simulink model "pressure"  (R2023b)
settings: Solver=FixedStepAuto  StartTime=0.0  StopTime=inf  RelTol=1e-3  EnableMultiTasking=on
PreLoadFcn:
  | a = 1;
InitFcn:
  | a = 1;
libraries: dspsigops x4, dspstat3 x3, simulink x2, bbblueSensorLib x1, dspfdesign x1
settings Model: SimulationMode=external  ExtModeTrigDuration=100  Creator=felih  LastModifiedBy=felih
settings SolverCC: PositivePriorityOrder=on
settings OptimizationCC: EnhancedBackFolding=on  PassReuseOutputArgsAs=Individual arguments  ZeroExternalMemoryAtStartup=off  ZeroInternalMemoryAtStartup=off  MaxStackSize=64  OptimizeBlockOrder=speed  DifferentSizesBufferReuse=on  OptimizationCustomize=off  EfficientTunableParamExpr=on
settings DebuggingCC: ParameterTunabilityLossMsg=error
settings HardwareCC: ProdBitPerPointer=32  ProdBitPerSizeT=32  ProdBitPerPtrDiffT=32  ProdLargestAtomicInteger=Long  ProdLargestAtomicFloat=Double  ProdWordSize=32  ProdHWDeviceType=ARM Compatible->ARM Cortex
settings SFSimCC: MATLABDynamicMemAlloc=off
settings RTWCC: Description=Embedded Coder  SystemTargetFile=ert.tlc  HardwareBoard=BeagleBone Blue  TLCOptions="-aInlineSetEventsForThisBaseRateFcn=TLC_FALSE -aSuppressMultiTaskScheduler=TLC_FALSE  -aRateBasedStepFcn=0"  TemplateMakefile=ert_default_tmf  Toolchain=GNU GCC BeagleBone Blue
settings CodeAppCC: ForceParamTrailComments=on  IgnoreCustomStorageClasses=off  OperatorAnnotations=on  SimulinkDataObjDesc=on  SFDataObjDesc=on  InsertBlockDesc=on
settings ERTTargetCC: SupportContinuousTime=on  SupportVariableSizeSignals=on  ExtMode=on  ExtModeMexArgs='192.168.7.2' 0 17725

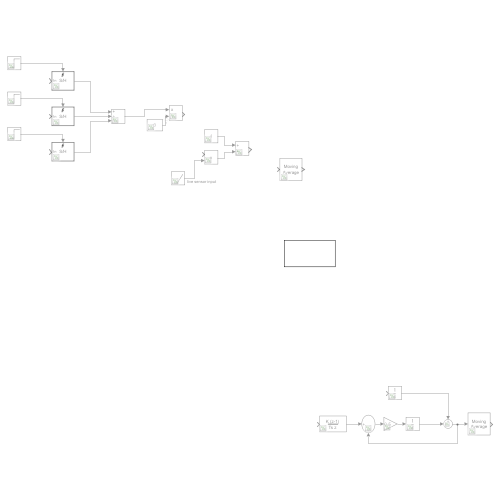
[thumbnail: Simulink's stored preview of the top-level diagram]
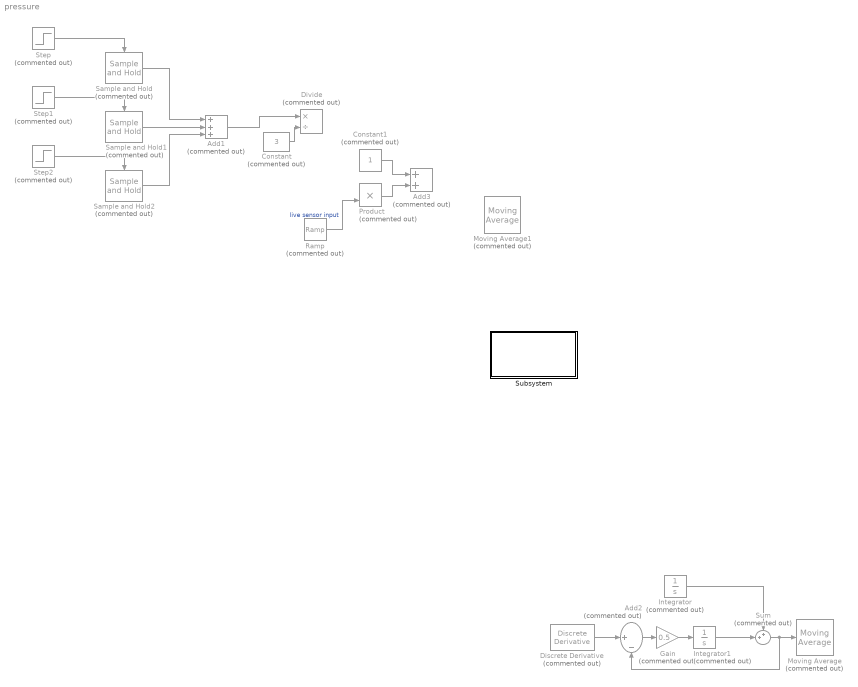
== system pressure ==
  Add1 : Sum  Commented=on  Inputs=+++
  Add2 : Sum  Commented=on  Inputs=|+-
  Add3 : Sum  Commented=on
  Constant : Constant  Commented=on  Value=3
  Constant1 : Constant  Commented=on
  Discrete Derivative : simulink/Discrete/Discrete Derivative  Commented=on  gainval=2  ICPrevScaledInput=0.0  OutMin=[]  OutMax=[]  OutDataType=fixdt(1, 16)  OutScaling=2^-10  DoSatur=off
  Divide : Product  Commented=on  Inputs=*/  RndMeth=Zero  SaturateOnIntegerOverflow=on
  Gain : Gain  Commented=on  Gain=0.5
  Integrator : Integrator  Commented=on
  Integrator1 : Integrator  Commented=on
  Moving Average : dspstat3/Moving Average  Commented=on  Method=Exponential weighting  ForgettingFactorPort=off  SpecifyWindowLength=on  WindowLength=10  OverlapLength=5  AllowArbitraryInputLength=off  ForgettingFactor=0.5  SimulateUsing=Code generation
  Moving Average1 : dspstat3/Moving Average  Commented=on  Method=Exponential weighting  ForgettingFactorPort=off  SpecifyWindowLength=on  WindowLength=10  OverlapLength=5  AllowArbitraryInputLength=on  ForgettingFactor=0.9  SimulateUsing=Code generation
  Product : Product  Commented=on
  Ramp : simulink/Sources/Ramp  Commented=on  slope=1  start=0  InitialOutput=0
  Sample and Hold : dspsigops/Sample and Hold  Commented=on  trig=Rising edge  initCond=0  latchinput=off
  Sample and Hold1 : dspsigops/Sample and Hold  Commented=on  trig=Rising edge  initCond=0  latchinput=off
  Sample and Hold2 : dspsigops/Sample and Hold  Commented=on  trig=Rising edge  initCond=0  latchinput=off
  Step : Step  Commented=on  SampleTime=0
  Step1 : Step  Commented=on  Time=1.1  SampleTime=0
  Step2 : Step  Commented=on  Time=0.9  SampleTime=0
  Subsystem : Subsystem
  Sum : Sum  Commented=on  Inputs=++|
  wires:
  Sample and Hold/1 -> Add1/1
  Sample and Hold1/1 -> Add1/2
  Step/1 -> Sample and Hold/Trigger
  Sample and Hold2/1 -> Add1/3
  Step1/1 -> Sample and Hold1/Trigger
  Step2/1 -> Sample and Hold2/Trigger
  Constant/1 -> Divide/2
  Add1/1 -> Divide/1
  Discrete Derivative/1 -> Add2/1
  Integrator1/1 -> Sum/2
  Integrator/1 -> Sum/1
  Add2/1 -> Gain/1
  Sum/1 -> Moving Average/1, Add2/2
  Gain/1 -> Integrator1/1
  Product/1 -> Add3/2
  Ramp/1 -> Product/2  "live sensor input"
  Constant1/1 -> Add3/1

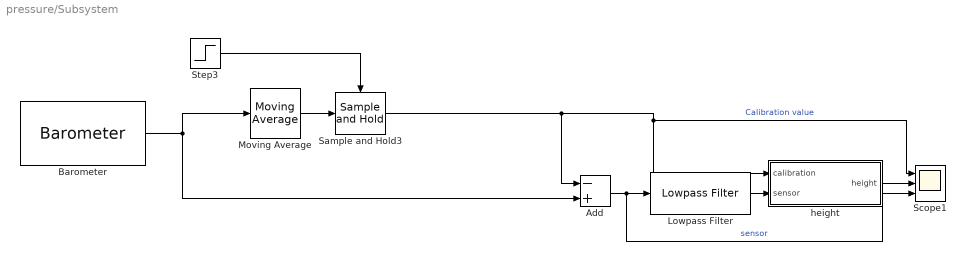
== system pressure/Subsystem ==
  Add : Sum  Inputs=-+
  Barometer : bbblueSensorLib/Barometer  OSRSelection=16  IIRFilterCoeff=2  SampleTime=0.01
  Lowpass Filter : dspfdesign/Lowpass Filter  FilterType=FIR  DesignForMinimumOrder=on  FilterOrder=50  PassbandFrequency=500  StopbandFrequency=800  PassbandRipple=0.1  StopbandAttenuation=80  SampleRateMode=Specify on dialog  SampleRate=44100  SimulateUsing=Interpreted execution  roundingMode=Floor  coeffsDataTypeStr=fixdt(1,16)
  Moving Average : dspstat3/Moving Average  Method=Exponential weighting  ForgettingFactorPort=off  SpecifyWindowLength=on  WindowLength=4  OverlapLength=3  AllowArbitraryInputLength=off  ForgettingFactor=1.0  SimulateUsing=Code generation
  Sample and Hold3 : dspsigops/Sample and Hold  trig=Rising edge  initCond=0  latchinput=off
  Scope1 : Scope  NumInputPorts=3
  Step3 : Step  Time=2  SampleTime=0
  height : MATLAB Function  TreatAsAtomicUnit=on
  wires:
  Add/1 -> Lowpass Filter/1, Scope1/3  "sensor"
  Barometer/1 -> Moving Average/1, Add/2
  Sample and Hold3/1 -> Scope1/1, height/1(calibration), Add/1  "Calibration value"
  Step3/1 -> Sample and Hold3/Trigger
  height/1(height) -> Scope1/2
  Moving Average/1 -> Sample and Hold3/1
  Lowpass Filter/1 -> height/2(sensor)

== matlab function pressure/Subsystem/height ==
  data: calibration input; sensor input; height output
function height = fcn(calibration,sensor)

% barometic formula

height = -(sensor/calibration)*8430 ;
